simulink model "ep4_4"  (R2018a)
settings: Solver=VariableStepAuto  StartTime=0.0  StopTime=100  MaxStep=0.001  RelTol=1e-3
values from neighbouring files (symbols this model uses):
  a1 = 1.3    [ep6_bungee.m]
  a2 = 1.1    [ep6_bungee.m]
  g = 9.8    [ep6_bungee.m]
  h = 80    [ep6_bungee.m]
  m = 70    [ep6_bungee.m]
  x0 = 30    [ep6_bungee.m]
undefined symbols (not defined in the file or in its folder): k
settings Model: Creator=zheny  LastModifiedBy=zheny

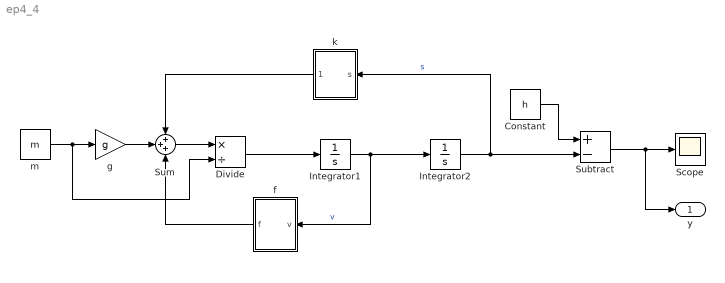
== system ep4_4 ==
  Constant : Constant  Value=h
  Divide : Product  Inputs=*/
  Integrator1 : Integrator
  Integrator2 : Integrator
  Scope : Scope
  Subtract : Sum  Inputs=+-
  Sum : Sum  Inputs=+++
  f : Subsystem  mask(空气阻力){a1=a1, a2=a2}
      mask help: -a1*v-a2*v*abs(v)
      mask Help:
      | 空气阻力
      | -a1*v-a2*v*abs(v)
      mask Display:
      | plot([0:0.01:1], [0:0.01:1].*[0:0.01:1])
      | port_label('input', 1, 'v')
      | port_label('output', 1, 'F')
  g : Gain  Gain=g
  k : Subsystem  mask(弹性力){k=k, x0=x0}
      mask help: -k(x-x0)
      mask Help:
      | 弹性力
      | -k(x-x0)
      mask Display:
      | plot([0:0.01:1], [0:0.01:1])
      | port_label('input', 1, 'S')
      | port_label('output', 1, 'K')
  m : Constant  Value=m
  y : Outport
  wires:
  Integrator2/1 -> Subtract/2, k/1(s)  "s"
  Integrator1/1 -> f/1(v), Integrator2/1  "v"
  m/1 -> Divide/2, g/1
  g/1 -> Sum/2
  Sum/1 -> Divide/1
  f/1(f) -> Sum/3
  k/1(Out1) -> Sum/1
  Constant/1 -> Subtract/1
  Subtract/1 -> y/1, Scope/1
  Divide/1 -> Integrator1/1

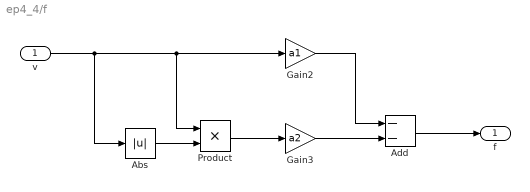
== system ep4_4/f ==
  v : Inport
  Abs : Abs
  Add : Sum  Inputs=--
  Gain2 : Gain  Gain=a1
  Gain3 : Gain  Gain=a2
  Product : Product
  f : Outport
  wires:
  Add/1 -> f/1
  Product/1 -> Gain3/1
  Abs/1 -> Product/2
  Gain3/1 -> Add/2
  Gain2/1 -> Add/1
  v/1 -> Abs/1, Product/1, Gain2/1

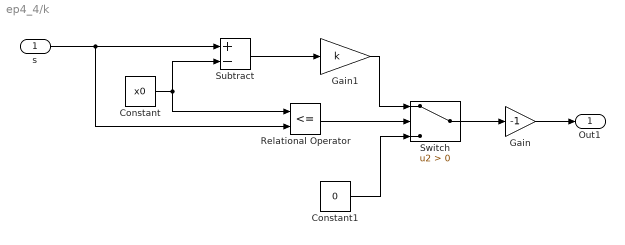
== system ep4_4/k ==
  s : Inport
  Constant : Constant  Value=x0
  Constant1 : Constant  Value=0
  Gain : Gain  Gain=-1
  Gain1 : Gain  Gain=k
  Relational Operator : RelationalOperator  Operator=<=  OutDataTypeStr=boolean  RndMeth=Simplest
  Subtract : Sum  Inputs=+-
  Switch : Switch  Criteria=u2 > Threshold
  Out1 : Outport
  wires:
  Gain1/1 -> Switch/1
  s/1 -> Subtract/1, Relational Operator/2
  Relational Operator/1 -> Switch/2
  Constant/1 -> Relational Operator/1, Subtract/2
  Constant1/1 -> Switch/3
  Subtract/1 -> Gain1/1
  Gain/1 -> Out1/1
  Switch/1 -> Gain/1
